simulink model "robusto"  (R2024a)
settings: Solver=VariableStepAuto  StartTime=0.0  StopTime=70  RelTol=1e-3
values from neighbouring files (symbols this model uses):
  Kd = diag([108 68 58 200])    [TRAIETTORIA.m]    (also in traiettoriafperfettadefinitiva1.m)
  KD = diag([1 1 1 1])    [TRAIETTORIA.m]    (also in traiettoriafperfettadefinitiva1.m = diag([1 1 1 1]*150))
  Kp = diag([13 13 11 1000])    [TRAIETTORIA.m]    (also in traiettoriafperfettadefinitiva1.m)
  KP = diag([1 1 1 1])    [TRAIETTORIA.m]    (also in traiettoriafperfettadefinitiva1.m = diag([1 1 1 1]*50))
  Q = lyap(H,P)    [TRAIETTORIA.m]    (also in traiettoriafperfettadefinitiva1.m)
undefined symbols (not defined in the file or in its folder): DiscIntNeverNeededParam
settings Model: Creator=ThinkPad  LastModifiedBy=UTENTE
settings ModelReferenceCC: EnableRefExpFcnMdlSchedulingChecks=on
settings RTWCC: GPUComputeCapability=3.5

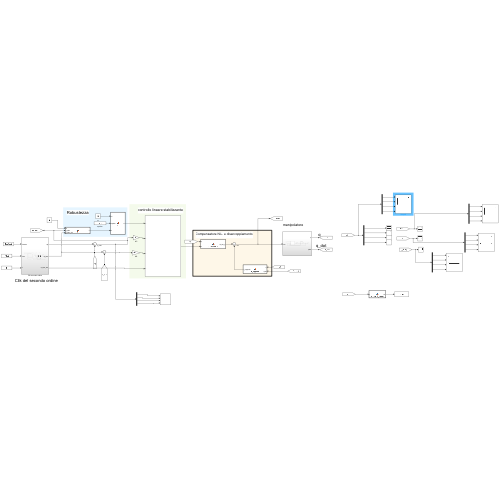
[thumbnail: Simulink's stored preview of the top-level diagram]
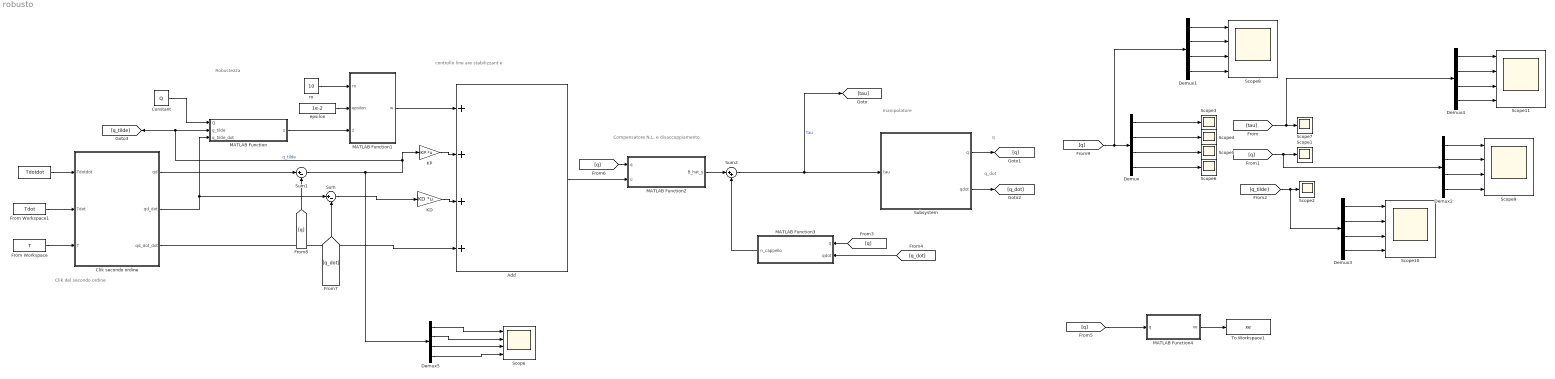
== system robusto ==
  note: controllo line are stabilizzant e
  note: q_dot
  note: Robustezza
  note: Clik del secondo ordine
  note: manipolatore
  note: Compensatore N.L. e disaccoppiamento
  note: q
  "   " : FromWorkspace  VariableName=Tdotdot
  Add : Sum  Inputs=++++
  Clik secondo ordine : Subsystem
  Constant : Constant  Value=Q
  Demux{,1..5} (6 alike) : Demux
  From Workspace : FromWorkspace  VariableName=T
  From Workspace1 : FromWorkspace  VariableName=Tdot
  KD : Gain  Gain=KD  Multiplication=Matrix(K*u)
  KP : Gain  Gain=KP  Multiplication=Matrix(K*u)
  MATLAB Function : MATLAB Function  TreatAsAtomicUnit=on
  MATLAB Function1 : MATLAB Function  TreatAsAtomicUnit=on
  MATLAB Function2 : MATLAB Function  TreatAsAtomicUnit=on
  MATLAB Function3 : MATLAB Function  TreatAsAtomicUnit=on
  MATLAB Function4 : MATLAB Function  TreatAsAtomicUnit=on
  Scope{,8..11} (5 alike) : Scope  NumInputPorts=4
  Scope{1..7} (7 alike) : Scope
  Subsystem : Subsystem
  Sum : Sum  Inputs=|+-
  Sum1 : Sum  Inputs=|+-
  Sum2 : Sum  Inputs=|++
  To Workspace1 : ToWorkspace  VariableName=xe  SampleTime=-1
  epsilon : Constant  Value=1e-2
  ro : Constant  Value=10
  wires:
  [tau] -> Demux4/1, Scope7/1
  MATLAB Function4/1(xe) -> To Workspace1/1
  Demux/3 -> Scope5/1
  Demux3/3 -> Scope10/3
  Demux3/1 -> Scope10/1
  [q_tilde] -> Demux3/1, Scope2/1
  Demux4/4 -> Scope11/4
  "   "/1 -> Clik secondo ordine/1(Tdotdot)
  [q] -> Demux2/1, Scope1/1
  KP/1 -> Add/2
  Demux/2 -> Scope4/1
  Subsystem/1(q) -> [q]
  Demux2/3 -> Scope9/3
  ro/1 -> MATLAB Function1/1(ro)
  MATLAB Function1/1(w) -> Add/1
  Demux2/1 -> Scope9/1
  Demux4/3 -> Scope11/3
  Demux3/2 -> Scope10/2
  Demux/1 -> Scope3/1
  Sum/1 -> KD/1
  From Workspace/1 -> Clik secondo ordine/3(T)
  Subsystem/2(qdot) -> [q_dot]
  Demux1/1 -> Scope8/1
  Sum1/1 -> Demux5/1, [q_tilde], MATLAB Function/2(q_tilde), KP/1  "q_tilde"
  Add/1 -> MATLAB Function2/2(u)
  Demux2/4 -> Scope9/4
  Demux1/3 -> Scope8/3
  epsilon/1 -> MATLAB Function1/2(epsilon)
  From Workspace1/1 -> Clik secondo ordine/2(Tdot)
  Demux3/4 -> Scope10/4
  Demux4/2 -> Scope11/2
  KD/1 -> Add/3
  Demux2/2 -> Scope9/2
  MATLAB Function3/1(n_cappello) -> Sum2/2
  MATLAB Function2/1(B_hat_y) -> Sum2/1
  MATLAB Function/1(z) -> MATLAB Function1/3(z)
  Demux/4 -> Scope6/1
  Clik secondo ordine/3(qd_dot_dot) -> Add/4
  Clik secondo ordine/1(qd) -> Sum1/1
  Demux4/1 -> Scope11/1
  Clik secondo ordine/2(qd_dot) -> MATLAB Function/3(q_tilde_dot), Sum/1
  Sum2/1 -> [tau], Subsystem/1(tau)  "tau"
  Demux1/2 -> Scope8/2
  Demux1/4 -> Scope8/4
  [q] -> MATLAB Function3/1(q)
  [q_dot] -> MATLAB Function3/2(qdot)
  [q] -> MATLAB Function4/1(q)
  [q] -> MATLAB Function2/1(q)
  [q_dot] -> Sum/2
  [q] -> Sum1/2
  [q] -> Demux1/1, Demux/1
  Constant/1 -> MATLAB Function/1(Q)
  Demux5/1 -> Scope/1
  Demux5/2 -> Scope/2
  Demux5/3 -> Scope/3
  Demux5/4 -> Scope/4

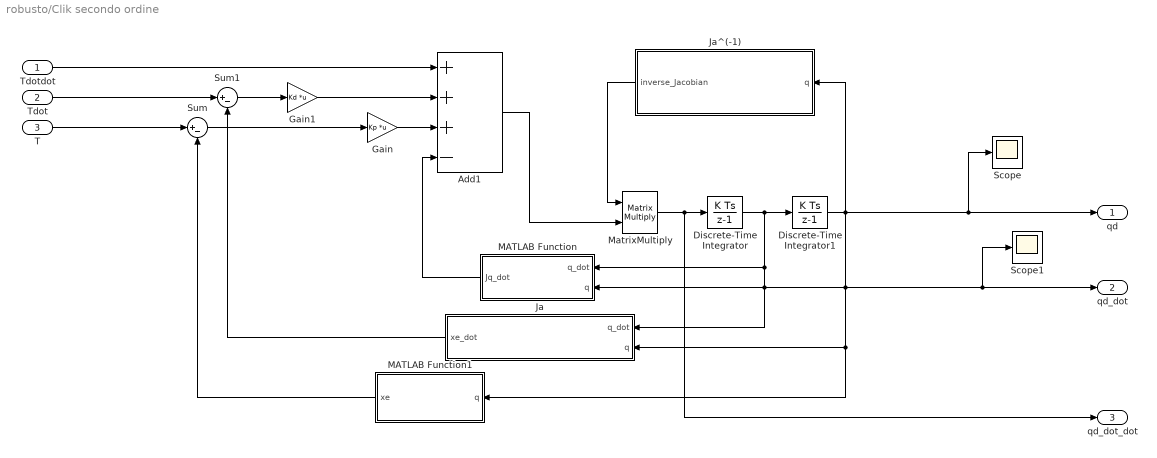
== system robusto/Clik secondo ordine ==
  Tdotdot : Inport
  Tdot : Inport  Port=2
  T : Inport  Port=3
  Add1 : Sum  Inputs=+++-
  Discrete-Time Integrator : DiscreteIntegrator  InitialCondition=[0 0 0 0]'  SampleTime=0.001  ICPrevOutput=DiscIntNeverNeededParam  ICPrevScaledInput=DiscIntNeverNeededParam
  Discrete-Time Integrator1 : DiscreteIntegrator  InitialCondition=[-0.2505, 0.6750, 0, 0.5]'  SampleTime=0.001  ICPrevOutput=DiscIntNeverNeededParam  ICPrevScaledInput=DiscIntNeverNeededParam
  Gain : Gain  Gain=Kp  Multiplication=Matrix(K*u)
  Gain1 : Gain  Gain=Kd  Multiplication=Matrix(K*u)
  Ja : MATLAB Function  TreatAsAtomicUnit=on
  Ja^(-1) : MATLAB Function  TreatAsAtomicUnit=on
  MATLAB Function : MATLAB Function  TreatAsAtomicUnit=on
  MATLAB Function1 : MATLAB Function  TreatAsAtomicUnit=on
  MatrixMultiply : Product  Multiplication=Matrix(*)
  Scope : Scope
  Scope1 : Scope
  Sum : Sum  Inputs=|+-
  Sum1 : Sum  Inputs=|+-
  qd : Outport
  qd_dot : Outport  Port=2
  qd_dot_dot : Outport  Port=3
  wires:
  Gain/1 -> Add1/3
  Gain1/1 -> Add1/2
  Add1/1 -> MatrixMultiply/2
  Discrete-Time Integrator1/1 -> Scope/1, qd/1, Ja/2(q), MATLAB Function1/1(q), MATLAB Function/2(q), Ja^(-1)/1(q)
  MATLAB Function1/1(xe) -> Sum/2
  MATLAB Function/1(Jq_dot) -> Add1/4
  Ja/1(xe_dot) -> Sum1/2
  Discrete-Time Integrator/1 -> Scope1/1, qd_dot/1, Ja/1(q_dot), MATLAB Function/1(q_dot), Discrete-Time Integrator1/1
  Sum1/1 -> Gain1/1
  Ja^(-1)/1(inverse_Jacobian) -> MatrixMultiply/1
  MatrixMultiply/1 -> qd_dot_dot/1, Discrete-Time Integrator/1
  Sum/1 -> Gain/1
  Tdot/1 -> Sum1/1
  Tdotdot/1 -> Add1/1
  T/1 -> Sum/1

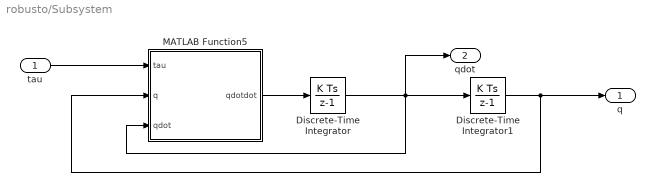
== system robusto/Subsystem ==
  tau : Inport
  Discrete-Time Integrator : DiscreteIntegrator  InitialCondition=[0 0 0 0]'  SampleTime=0.001  ICPrevOutput=DiscIntNeverNeededParam  ICPrevScaledInput=DiscIntNeverNeededParam
  Discrete-Time Integrator1 : DiscreteIntegrator  InitialCondition=[pi/2 pi/3 pi/5 0.5]'  SampleTime=0.001  ICPrevOutput=DiscIntNeverNeededParam  ICPrevScaledInput=DiscIntNeverNeededParam
  MATLAB Function5 : MATLAB Function  TreatAsAtomicUnit=on
  q : Outport
  qdot : Outport  Port=2
  wires:
  MATLAB Function5/1(qdotdot) -> Discrete-Time Integrator/1
  tau/1 -> MATLAB Function5/1(tau)
  Discrete-Time Integrator1/1 -> q/1, MATLAB Function5/2(q)
  Discrete-Time Integrator/1 -> qdot/1, Discrete-Time Integrator1/1, MATLAB Function5/3(qdot)

== matlab function robusto/MATLAB Function4 ==
  data: q input; xe output
function xe = cinematica_diretta(q)
% T_4_0=[cos(q(4))*(cos(q(1))*cos(q(2))-sin(q1)*sin(q2))+sin(q(4))*(cos(q1)*sin(q(2))+cos(q(2))*sin(q(1)))   cos(q(4))*(cos(q(1))*sin(q(2))+cos(q(2))*sin(q(1)))-sin(q(4))*(cos(q(1))*cos(q(2))-sin(q(1))*sin(q(2)))  0 cos(q(1))/2+(cos(q(1))*cos(q(2)))/2-(sin(q(1))*sin(q(2)))/2;
%         cos(q(4))*(cos(q(1))*sin(q(2))+cos(q(2))*sin(q(1)))-sin(q(4))*(cos(q(1))*cos(q(2))-sin(q(1))*sin(q(2))) -cos(q(4))*(cos(q(1))*cos(q(2))-sin(q(1))*sin(q(2)))-sin(q(4))*(cos(q(1))*sin(q(2))+cos(q(2))*sin(q(1)))  0 sin(q(1))/2+(cos(q(1))*sin(q(2)))/2+(cos(q(2))*sin(q(2)))/2;
%                       0                                                      0                    -1                                                1-q(3);
%         0                                       0                                         0                                                                                                                                      1];

x_e=[0.5*cos(q(1))+0.5*cos(q(1)+q(2));
    0.5*sin(q(1))+0.5*sin(q(1)+q(2));
        1-q(3);
        q(1)+q(2)-q(4)];
xe=x_e;
end

== matlab function robusto/Clik secondo ordine/Ja ==
  data: q_dot input; q input; xe_dot output
function xe_dot = xe_dot(q_dot, q)

J=[-0.5*sin(q(1))-0.5*sin(q(1)+q(2)) -0.5*sin(q(1)+q(2)) 0 0;
    0.5*cos(q(1))+0.5*cos(q(1)+q(2)) 0.5*cos(q(1)+q(2)) 0 0;
    0 0 -1 0;
    1 1 0 -1];
xe_dot=J*q_dot;
end

== matlab function robusto/Clik secondo ordine/MATLAB Function ==
  data: q_dot input; q input; Jq_dot output
function Jq_dot = Jq_dot(q_dot, q)
J_dot=[-0.5*cos(q(1))*q_dot(1)-0.5*cos(q(1)+q(2))*(q_dot(1)+q_dot(2)) -0.5*cos(q(1)+q(2))*(q_dot(1)+q_dot(2)) 0 0;
    -0.5*sin(q(1))*q_dot(1)-0.5*sin(q(1)+q(2))*(q_dot(1)+q_dot(2)) -0.5*sin(q(1)+q(2))*(q_dot(1)+q_dot(2)) 0 0;
    0 0 0 0;
    0 0 0 0];
Jq_dot=J_dot*q_dot;
end

== matlab function robusto/Clik secondo ordine/MATLAB Function1 ==
  data: q input; xe output
function xe = cinematica_diretta(q)
% T_4_0=[cos(q(4))*(cos(q(1))*cos(q(2))-sin(q1)*sin(q2))+sin(q(4))*(cos(q1)*sin(q(2))+cos(q(2))*sin(q(1)))   cos(q(4))*(cos(q(1))*sin(q(2))+cos(q(2))*sin(q(1)))-sin(q(4))*(cos(q(1))*cos(q(2))-sin(q(1))*sin(q(2)))  0 cos(q(1))/2+(cos(q(1))*cos(q(2)))/2-(sin(q(1))*sin(q(2)))/2;
%         cos(q(4))*(cos(q(1))*sin(q(2))+cos(q(2))*sin(q(1)))-sin(q(4))*(cos(q(1))*cos(q(2))-sin(q(1))*sin(q(2))) -cos(q(4))*(cos(q(1))*cos(q(2))-sin(q(1))*sin(q(2)))-sin(q(4))*(cos(q(1))*sin(q(2))+cos(q(2))*sin(q(1)))  0 sin(q(1))/2+(cos(q(1))*sin(q(2)))/2+(cos(q(2))*sin(q(2)))/2;
%                       0                                                      0                    -1                                                1-q(3);
%         0                                       0                                         0                                                                                                                                      1];

x_e=[0.5*cos(q(1))+0.5*cos(q(1)+q(2));
    0.5*sin(q(1))+0.5*sin(q(1)+q(2));
        1-q(3);
        q(1)+q(2)-q(4)];
xe=x_e;
end

== matlab function robusto/MATLAB Function ==
  data: Q input; q_tilde input; z output; q_tilde_dot input
function z = z(Q, q_tilde, q_tilde_dot)
D=[zeros(4,4);
   eye(4)];


%Q=diag([1 1 100 1 0.1 0.1 10 0.1]);
% Q=diag([.1 .1 .1 100 1 1 1 100]);
z=(D')*Q*[q_tilde; q_tilde_dot];
end

== matlab function robusto/MATLAB Function1 ==
  data: ro input; epsilon input; z input; w output
function w = w(ro, epsilon, z)

norma_z=norm(z);

if norma_z > epsilon 
    w=ro*z/norma_z;
else
    w=ro*z/epsilon;
end

end

== matlab function robusto/MATLAB Function2 ==
  data: q input; u input; B_hat_y output
function B_hat_y = B_cappello_y(q, u)
d0=1;
a1=0.5;
a2=0.5;
l1=0.25;
l2=0.25;
ml1=20;
ml2=20;
ml3=10;
ml4=0;
Il1=4;
Il2=4;
Il3=0;
Il4=1;
kr1=1;
kr2=1;
kr3=50;
kr4=20;
Im1=0,01;
Im2=0,01;
Im3=0,005;
Im4=0,001;
Fm1=0.00005;
Fm2=0.00005;
Fm3=0.01;
Fm4=0.005;
%ml=3;
mm1=0;
mm2=0;
mm3=0;
mm4=0;

Jp_l1=[-l1*sin(q(1)) 0 0  0;
        l1*cos(q(1)) 0 0  0;
        0            0 0  0];
    
Jo_l1=[0 0 0 0;
       0 0 0 0;
       1 0 0 0];
   
Jp_l2=[-a1*sin(q(1))-l2*sin(q(1)+q(2)) -l2*sin(q(1)+q(2)) 0  0;
        a1*cos(q(1))+l2*cos(q(1)+q(2)) +l2*cos(q(1)+q(2)) 0  0;
        0                                      0          0  0];
   
Jo_l2=[0 0 0 0;
       0 0 0 0;
       1 1 0 0];

Jp_l3=[-a1*sin(q(1))-a2*sin(q(1)+q(2)) -a2*sin(q(1)+q(2))  0   0;
        a1*cos(q(1))+a2*cos(q(1)+q(2)) +a2*cos(q(1)+q(2))  0   0;
        0                                               0  -1  0];
Jo_l3=[0 0 0 0;
       0 0 0 0;
       1 1 0 0];
 
Jp_l4=[-a1*sin(q(1))-a2*sin(q(1)+q(2)) -a2*sin(q(1)+q(2))  0   0;
        a1*cos(q(1))+a2*cos(q(1)+q(2)) +a2*cos(q(1)+q(2))  0   0;
        0                                               0  -1  0];
Jo_l4=[0 0 0 0;
       0 0 0 0;
       1 1 0 -1];

Jp_m1=[0 0 0 0;
       0 0 0 0;
       0 0 0 0];
   
Jo_m1=[0 0 0 0;
       0 0 0 0;
       kr1 0 0 0];

Jp_m2=[-a1*sin(q(1)) 0 0 0;
       a1*cos(q(1)) 0 0 0;
           0        0 0 0];
       
Jo_m2=[0 0 0 0;
       0 0 0 0;
       1 kr2 0 0];

Jp_m3=[-a1*sin(q(1))-a2*sin(q(1)+q(2)) -a2*sin(q(1)+q(2))  0 0;
        a1*cos(q(1))+a2*cos(q(1)+q(2)) +a2*cos(q(1)+q(2))  0 0;
                      0                         0          0 0];

Jo_m3=[0 0 0 0;
       0 0 0 0;
       1 1 -kr3 0];

Jp_m4=[-a1*sin(q(1))-a2*sin(q(1)+q(2)) -a2*sin(q(1)+q(2))  0 0;
        a1*cos(q(1))+a2*cos(q(1)+q(2)) +a2*cos(q(1)+q(2))  0 0;
                      0                         0          -1 0];
Jo_m4=[0 0 0 0;
       0 0 0 0;
       1 1 0 -kr4];

B1=ml1*(Jp_l1')*Jp_l1+(Jo_l1')*Il1*Jo_l1+mm1*(Jp_m1')*Jp_m1+(Jo_m1')*Im1*Jo_m1;
B2=ml2*(Jp_l2')*Jp_l2+(Jo_l2')*Il2*Jo_l2+mm2*(Jp_m2')*Jp_m2+(Jo_m2')*Im2*Jo_m2;
B3=ml3*(Jp_l3')*Jp_l3+(Jo_l3')*Il3*Jo_l3+mm3*(Jp_m3')*Jp_m3+(Jo_m3')*Im3*Jo_m3;
B4=(ml4)*(Jp_l4')*Jp_l4+(Jo_l4')*Il4*Jo_l4+mm4*(Jp_m4')*Jp_m4+(Jo_m4')*Im4*Jo_m4;

B=B1+B2+B3+B4;
B_hat=[B(1,1) 0 0 0;
0 B(2,2) 0 0;
0 0 B(3,3) 0;
0 0 0 B(4,4)];
B_hat_y = B*u;
end

== matlab function robusto/MATLAB Function3 ==
  data: q input; n_cappello output; qdot input
function n_cappello = n_cappello(q, qdot)
d0=1;
a1=0.5;
a2=0.5;
l1=0.25;
l2=0.25;
ml1=20;
ml2=20;
ml3=10;
Il1=4;
Il2=4;
Il4=1;
kr1=1;
kr2=1;
kr3=50;
kr4=20;
Im1=0,01;
Im2=0,01;
Im3=0,005;
Im4=0,001;
Fm1=0.00005;
Fm2=0.00005;
Fm3=0.01;
Fm4=0.005;
%ml=3;
mm1=0;
mm2=0;
mm3=0;
mm4=0;

Jp_l1=[-l1*sin(q(1)) 0 0  0;
        l1*cos(q(1)) 0 0  0;
        0            0 0  0];
    
Jo_l1=[0 0 0 0;
       0 0 0 0;
       1 0 0 0];
   
Jp_l2=[-a1*sin(q(1))-l2*sin(q(1)+q(2)) -l2*sin(q(1)+q(2)) 0  0;
        a1*cos(q(1))+l2*cos(q(1)+q(2)) +l2*cos(q(1)+q(2)) 0  0;
        0                                      0          0  0];
   
Jo_l2=[0 0 0 0;
       0 0 0 0;
       1 1 0 0];

Jp_l3=[-a1*sin(q(1))-a2*sin(q(1)+q(2)) -a2*sin(q(1)+q(2))  0   0;
        a1*cos(q(1))+a2*cos(q(1)+q(2)) +a2*cos(q(1)+q(2))  0   0;
        0                                               0  -1  0];
Jo_l3=[0 0 0 0;
       0 0 0 0;
       1 1 0 0];
 
Jp_l4=[-a1*sin(q(1))-a2*sin(q(1)+q(2)) -a2*sin(q(1)+q(2))  0   0;
        a1*cos(q(1))+a2*cos(q(1)+q(2)) +a2*cos(q(1)+q(2))  0   0;
        0                                               0  -1  0];
Jo_l4=[0 0 0 0;
       0 0 0 0;
       1 1 0 -1];

Jp_m1=[0 0 0 0;
       0 0 0 0;
       0 0 0 0];
   
Jo_m1=[0 0 0 0;
       0 0 0 0;
       kr1 0 0 0];

Jp_m2=[-a1*sin(q(1)) 0 0 0;
       a1*cos(q(1)) 0 0 0;
           0        0 0 0];
       
Jo_m2=[0 0 0 0;
       0 0 0 0;
       1 kr2 0 0];

Jp_m3=[-a1*sin(q(1))-a2*sin(q(1)+q(2)) -a2*sin(q(1)+q(2))  0 0;
        a1*cos(q(1))+a2*cos(q(1)+q(2)) +a2*cos(q(1)+q(2))  0 0;
                      0                         0          0 0];

Jo_m3=[0 0 0 0;
       0 0 0 0;
       1 1 -kr3 0];

Jp_m4=[-a1*sin(q(1))-a2*sin(q(1)+q(2)) -a2*sin(q(1)+q(2))  0 0;
        a1*cos(q(1))+a2*cos(q(1)+q(2)) +a2*cos(q(1)+q(2))  0 0;
                      0                         0          -1 0];
Jo_m4=[0 0 0 0;
       0 0 0 0;
       1 1 0 -kr4];


Fv=diag([kr1^2*Fm1 kr2^2*Fm2 kr3^2*Fm3 kr4^2*Fm4]);
% Fv=[Fm1 0   0   0;
%     0   Fm2 0   0;
%     0   0   Fm3 0;
%     0   0   0   Fm4];

g=[0 0 -9.81*(ml3) 0]';

Jpl1_dq1=[-l1*cos(q(1)) 0 0 0;
    -l1*sin(q(1)) 0 0 0;
    0 0 0 0];

Jpl2_dq1=[-a1*cos(q(1))-l2*cos(q(1)+q(2)) -l2*cos(q(1)+q(2)) 0 0;
    -a1*sin(q(1))-l2*sin(q(1)+q(2)) -l2*sin(q(1)+q(2)) 0 0;
    0 0 0 0];

Jpl2_dq2=[-a2*cos(q(1)+q(2)) -a2*cos(q(1)+q(2)) 0 0;
    -a2*sin(q(1)+q(2)) -a2*sin(q(1)+q(2)) 0 0;
    0 0 0 0];

Jpl4_dq1=[-a1*cos(q(1))-a2*cos(q(1)+q(2)) -a2*cos(q(1)+q(2)) 0 0;
    -a1*sin(q(1))-a2*sin(q(1)+q(2)) -a2*sin(q(1)+q(2)) 0 0;
    0 0 0 0];

Jpl4_dq2=[-a2*sin(q(1)+q(2)) -a2*sin(q(1)+q(2)) 0 0;
    -a2*cos(q(1)+q(2)) -a2*cos(q(1)+q(2)) 0 0;
    0 0 0 0];

dBdq1=ml1*(Jpl1_dq1'*Jp_l1+Jp_l1'*Jpl1_dq1)+ml2*(Jpl2_dq1'*Jp_l2+Jp_l2'*Jpl2_dq1)...
    +ml3*(Jpl4_dq1'*Jp_l4+Jp_l4'*Jpl4_dq1);

dBdq2=ml2*(Jpl2_dq2'*Jp_l2+Jp_l2'*Jpl2_dq2)+ml3*(Jpl4_dq2'*Jp_l4+Jp_l4'*Jpl4_dq2);

H=zeros(4,4,4);


for i=1:4
    for j=1:4
        for k=1:4
            H(i,j,k)=0;
        end
    end
end

H(1,1,2)=1/2*(dBdq2(1,1)+dBdq1(1,2)-dBdq1(1,2));
H(1,2,1)=H(1,1,2); 
H(1,2,2)=1/2*(dBdq2(1,2)+dBdq2(1,2)-dBdq1(2,2));
H(2,1,1)=1/2*(dBdq1(2,1)+dBdq1(2,1)-dBdq2(1,1));
H(2,1,2)=1/2*(dBdq2(2,1)+dBdq1(2,2)-dBdq2(1,2));
H(2,2,1)=H(2,1,2);
H(2,2,2)=1/2*(dBdq2(2,2)+dBdq2(2,2)-dBdq2(2,2));

C=zeros(4,4);
for i=1:4
    for j=1:4
        C(i,j)=0;
    end
end

for i=1:4
    for j=1:4
        for k=1:4
            r=H(i,j,k)*qdot(k);
            C(i,j)=C(i,j)+r;
        end
    end
end

n_cappello=C*qdot+Fv*qdot+g;

end

== matlab function robusto/Subsystem/MATLAB Function5 ==
  data: tau input; q input; qdot input; qdotdot output
function qdotdot = fcn(tau, q, qdot)
  
    d0=1; %m
    a1=0.5; %m
    a2=0.5; %m
    
    l1=0.25; %m
    l2=0.25; %m
    ml1=20; %kg
    ml2=20; %kg
    ml3=10; %kg
    ml4=0; %kg
    Il1=4; %kg�m2
    Il2=4; %kg�m2
    Il3=0;
    Il4=1; %kg�m2
    Kr1=1;
    Kr2=1;
    Kr3=50; %rad/m
    Kr4 =20;
    Im1=0.01; %kg�m2
    Im2=0.01; %kg�m2
    Im3=0.005; %kg�m2
    Im4=0.001;%kg
    Fm1=0.00005; %N�m�s/rad
    Fm2=0.00005; %N�m�s/rad
    Fm3=0.01; %N�m�s/rad
    Fm4 =0.005; %N�m�s/rad
    mm1=0;
    mm2=0;
    mm3=0;
    mm4=0;
    ml=3;
    
    Jp_l1=[-l1*sin(q(1)) 0 0 0; 
            l1*cos(q(1)) 0 0 0; 
            0 0 0 0];
    Jo_l1=[zeros(2,4)
           1 0 0 0];
    
    Jp_l2=[-a1*sin(q(1))-l2*sin(q(1)+q(2)) -l2*sin(q(1)+q(2)) 0 0; 
            a1*cos(q(1))+l2*cos(q(1)+q(2)) l2*cos(q(1)+q(2)) 0 0;
            0 0 0 0];
    Jo_l2=[zeros(2,4)
           1 1 0 0];
    
    Jp_l3=[-a1*sin(q(1))-a2*sin(q(1)+q(2)) -a2*sin(q(1)+q(2)) 0 0; 
            a1*cos(q(1))+a2*cos(q(1)+q(2)) a2*cos(q(1)+q(2)) 0 0;
            0 0 -1 0];
    Jo_l3 = [zeros(2,4)
             1 1 0 0];
    
    Jp_l4=Jp_l3;
    Jo_l4 = [zeros(2,4)
             1 1 0 -1];
    
    Jp_m1 = [0 0 0 0;
             0 0 0 0;
             0 0 0 0];
    Jo_m1 = [zeros(2,4)
             Kr1 0 0 0];
    
    Jp_m2 = [-a1*sin(q(1)) 0 0 0; 
            a1*cos(q(1)) 0 0 0; 
            0 0 0 0];
    Jo_m2 = [zeros(2,4)
             1 Kr2 0 0];
    
    Jp_m3 = [-a1*sin(q(1))-a2*sin(q(1)+q(2)) -a2*sin(q(1)+q(2)) 0 0; 
              a1*cos(q(1))+a2*cos(q(1)+q(2)) a2*cos(q(1)+q(2)) 0 0;
              0 0 0 0];
    Jo_m3 = [zeros(2,4)
             1 1 -Kr3 0];
    
    Jp_m4 = [-a1*sin(q(1))-a2*sin(q(1)+q(2)) -a2*sin(q(1)+q(2)) 0 0; 
              a1*cos(q(1))+a2*cos(q(1)+q(2)) a2*cos(q(1)+q(2)) 0 0;
              0 0 -1 0];
    Jo_m4 = [zeros(2,4)
             1 1 0 -Kr4];
    B1 = ml1*Jp_l1'*Jp_l1+Jo_l1'*Il1*Jo_l1+mm1*Jp_m1'*Jp_m1+Jo_m1'*Im1*Jo_m1;
    B2 = ml2*Jp_l2'*Jp_l2+Jo_l2'*Il2*Jo_l2+mm2*Jp_m2'*Jp_m2+Jo_m2'*Im2*Jo_m2;
    B3 = ml3*Jp_l3'*Jp_l3+Jo_l3'*Il3*Jo_l3+mm3*Jp_m3'*Jp_m3+Jo_m3'*Im3*Jo_m3;
    B4 = (ml4+ml)*Jp_l4'*Jp_l4+Jo_l4'*Il4*Jo_l4+mm4*Jp_m4'*Jp_m4+Jo_m4'*Im4*Jo_m4;
    B = B1+B2+B3+B4;
    
    Fv = diag([Kr1^2*Fm1 Kr2^2*Fm2 Kr3^2*Fm3 Kr4^2*Fm4]);
    g=[0 0 -9.81*(ml+ml3) 0]';
    
    Jpl1_dq1=[-l1*cos(q(1)) 0 0 0;
    -l1*sin(q(1)) 0 0 0;
    0 0 0 0];

Jpl2_dq1=[-a1*cos(q(1))-l2*cos(q(1)+q(2)) -l2*cos(q(1)+q(2)) 0 0;
    -a1*sin(q(1))-l2*sin(q(1)+q(2)) -l2*sin(q(1)+q(2)) 0 0;
    0 0 0 0];

Jpl2_dq2=[-a2*cos(q(1)+q(2)) -a2*cos(q(1)+q(2)) 0 0;
    -a2*sin(q(1)+q(2)) -a2*sin(q(1)+q(2)) 0 0;
    0 0 0 0];

Jpl4_dq1=[-a1*cos(q(1))-a2*cos(q(1)+q(2)) -a2*cos(q(1)+q(2)) 0 0;
    -a1*sin(q(1))-a2*sin(q(1)+q(2)) -a2*sin(q(1)+q(2)) 0 0;
    0 0 0 0];

Jpl4_dq2=[-a2*sin(q(1)+q(2)) -a2*sin(q(1)+q(2)) 0 0;
    -a2*cos(q(1)+q(2)) -a2*cos(q(1)+q(2)) 0 0;
    0 0 0 0];

% Calcolo matrice differenziate rispetto a dq1 dq2
dBdq1=ml1*(Jpl1_dq1'*Jp_l1+Jp_l1'*Jpl1_dq1)+ml2*(Jpl2_dq1'*Jp_l2+Jp_l2'*Jpl2_dq1)...
    +ml3*(Jpl4_dq1'*Jp_l4+Jp_l4'*Jpl4_dq1);

dBdq2=ml2*(Jpl2_dq2'*Jp_l2+Jp_l2'*Jpl2_dq2)+ml3*(Jpl4_dq2'*Jp_l4+Jp_l4'*Jpl4_dq2);

H=zeros(4,4,4);

% Inizializzazione simboli cristoffel del primo tipo
for i=1:4
    for j=1:4
        for k=1:4
            H(i,j,k)=0;
        end
    end
end

H(1,1,2)=1/2*(dBdq2(1,1)+dBdq1(1,2)-dBdq1(1,2));
H(1,2,1)=H(1,1,2); 
H(1,2,2)=1/2*(dBdq2(1,2)+dBdq2(1,2)-dBdq1(2,2));
H(2,1,1)=1/2*(dBdq1(2,1)+dBdq1(2,1)-dBdq2(1,1));
H(2,1,2)=1/2*(dBdq2(2,1)+dBdq1(2,2)-dBdq2(1,2));
H(2,2,1)=H(2,1,2);
H(2,2,2)=1/2*(dBdq2(2,2)+dBdq2(2,2)-dBdq2(2,2));


% C=sym('C',[4,4]);
C=zeros(4,4);
for i=1:4
    for j=1:4
        C(i,j)=0;
    end
end

% qdot=sym('qdot',[4,1]);

for i=1:4
    for j=1:4
        for k=1:4
            r=H(i,j,k)*qdot(k);
            C(i,j)=C(i,j)+r;
        end
    end
end
    
qdotdot = inv(B)*(tau-C*qdot-Fv*qdot-g);
end

== matlab function robusto/Clik secondo ordine/Ja^(-1) ==
  data: q input; inverse_Jacobian output
function inverse_Jacobian= i_j(q)

J=[-0.5*sin(q(1))-0.5*sin(q(1)+q(2)) -0.5*sin(q(1)+q(2)) 0 0;
    0.5*cos(q(1))+0.5*cos(q(1)+q(2)) 0.5*cos(q(1)+q(2)) 0 0;
    0 0 -1 0;
    1 1 0 -1];

J_inv=inv(J);

 inverse_Jacobian=J_inv;
end
